simulink model "eVTOL"  (R2025b)
settings: Solver=ode45  StartTime=0.0  StopTime=7  MaxStep=1e-4  RelTol=1e-3
InitFcn:
  | load('inner_controller_design.mat')
  | load('outer_controller_design.mat')
  | load('speed_controller_design.mat')
  | load('position_controller_design.mat')
  | load('tita_controller_design.mat')
values from neighbouring files (symbols this model uses):
  b = 1e-4    (= 0.0001)    [LE_final.m]    (also in outer_controller_design.mat)
  denC = [Kc*Tcontrolador,1]    [LI_final.m]    (also in inner_controller_design.mat = [0.0127388535032 1])
  J_motor = 0.01*(0.432^2)*2    (= 0.00373248)    [LE_final.m]    (also in outer_controller_design.mat)
  J_xz = 3.25    [angular_speed_controller_design.mat]    (also in tita_controller_design.mat = 2.16666666667)
  K_pos_den = [1 2.17655923708]    [position_controller_design.mat]
  K_pos_num = [0 1.57913670417]    [position_controller_design.mat]
  Ke = 1 / Kv_rad_per_V    (= 0.0347247148564)    [LE_final.m]    (also in outer_controller_design.mat)
  KF = 0.000504745724606    [speed_controller_design.mat]
  Ki = K * z    [LE_final.m]    (also in outer_controller_design.mat = 13312.7522358)
  Kp = K    [LE_final.m]    (also in outer_controller_design.mat = 52.8005114253)
  kQ = alpha_rpm * rpm2rad^-2    (= 1.07603097028e-05)    [LE_final.m]    (also in outer_controller_design.mat)
  Kt = 1*Ke    (= 0.0347247148564)    [LE_final.m]    (also in outer_controller_design.mat)
  Ktita_den = [1 61.1449635422]    [tita_controller_design.mat]
  Ktita_num = [1557.79440274 15875.2136603]    [tita_controller_design.mat]
  Kv_den = 1    [speed_controller_design.mat]
  Kv_num = 65.3451271947    [speed_controller_design.mat]
  l = 0.3    [speed_controller_design.mat]
  l_palanca = 0.4    [tita_controller_design.mat]
  La = 0.0004    [LI_final.m]    (also in inner_controller_design.mat)
  m = 13    [speed_controller_design.mat]
  numC = [Tcontrolador,1]    [LI_final.m]    (also in inner_controller_design.mat = [0.00398089171975 1])
  Ra = 0.066    [LI_final.m]    (also in inner_controller_design.mat)
libraries: slpidlib x5, simulink_extras x4
(part 2 of 2)

== matlab function eVTOL/Controlador de Posición y Velocidad/Motor Speed Calculator/Motor 3/MATLAB Function ==
  data: omega input; T_a output; kQ input; b input
function T_a = fcn(omega,kQ, b)
T_a=(omega^2)*kQ+b*omega; 
end
